simulink model "openMHA_test_ar_filter"  (R2020a)
settings: Solver=VariableStepAuto  StartTime=0.0  StopTime=stop_time  RelTol=1e-3
InitFcn:
  | test_ar_filter_init
StopFcn:
  | test_ar_filter_stop
values from neighbouring files (symbols this model uses):
  c1_a = exp( -1.0/(tau_a * fs) )    [test_FFT_to_gain_init.m]    (also in test_ar_filter_gaintable_init.m; test_ar_filter_init.m; test_db_ar_gaintable_init.m)
  c1_r = exp( -1.0/(tau_r * fs) )    [test_FFT_to_gain_init.m]    (also in test_ar_filter_gaintable_init.m; test_ar_filter_init.m; test_db_ar_gaintable_init.m)
  c2_a = 1.0 - c1_a    [test_FFT_to_gain_init.m]    (also in test_ar_filter_gaintable_init.m; test_ar_filter_init.m; test_db_ar_gaintable_init.m)
  c2_r = 1.0 - c1_r    [test_FFT_to_gain_init.m]    (also in test_ar_filter_gaintable_init.m; test_ar_filter_init.m; test_db_ar_gaintable_init.m)
libraries: simulink x1, dspsrcs4 x1
settings Model: PacingRate=112  Creator=t96f346  LastModifiedBy=t96f346

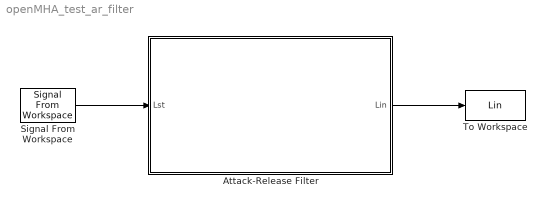
== system openMHA_test_ar_filter ==
  Attack-Release Filter : Subsystem
  Signal From Workspace : dspsrcs4/Signal From Workspace  X=Lst  Ts=1  nsamps=1  OutputAfterFinalValue=Setting to zero  ignoreOrWarnInputAndFrameLengths=off  OutputFrames=off
  To Workspace : ToWorkspace  VariableName=Lin  SampleTime=-1
      settings: Save2DSignal=2-D array (concatenate along first dimension)
  wires:
  Signal From Workspace/1 -> Attack-Release Filter/1(Lst)
  Attack-Release Filter/1(Lin) -> To Workspace/1

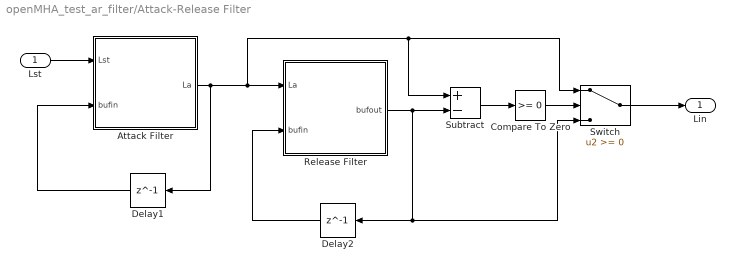
== system openMHA_test_ar_filter/Attack-Release Filter ==
  Lst : Inport
  Attack Filter : Subsystem  TreatAsAtomicUnit=on
  Compare To Zero : simulink/Logic and Bit Operations/Compare To Zero  relop=>=  OutDataTypeStr=boolean
  Delay1 : Delay  DelayLength=1  InitialCondition=65
  Delay2 : Delay  DelayLength=1  InitialCondition=65
  Release Filter : Subsystem  TreatAsAtomicUnit=on
  Subtract : Sum  Inputs=+-  OutDataTypeStr=Inherit: Same as accumulator
  Switch : Switch
  Lin : Outport  VectorParamsAs1DForOutWhenUnconnected=off
  wires:
  Lst/1 -> Attack Filter/1(Lst)
  Delay2/1 -> Release Filter/2(bufin)
  Delay1/1 -> Attack Filter/2(bufin)
  Subtract/1 -> Compare To Zero/1
  Switch/1 -> Lin/1
  Release Filter/1(bufout) -> Subtract/2, Delay2/1, Switch/3
  Compare To Zero/1 -> Switch/2
  Attack Filter/1(La) -> Delay1/1, Subtract/1, Switch/1, Release Filter/1(La)

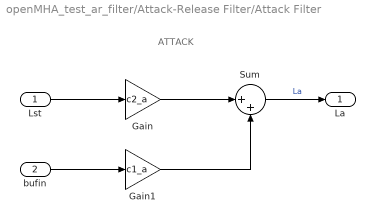
== system openMHA_test_ar_filter/Attack-Release Filter/Attack Filter ==
  note: ATTACK
  Lst : Inport
  bufin : Inport  Port=2
  Gain : Gain  Gain=c2_a
  Gain1 : Gain  Gain=c1_a
  Sum : Sum  Inputs=|++
  La : Outport  InitialOutput=0  VectorParamsAs1DForOutWhenUnconnected=off
  wires:
  Lst/1 -> Gain/1
  Gain/1 -> Sum/1
  Sum/1 -> La/1  "La"
  bufin/1 -> Gain1/1
  Gain1/1 -> Sum/2

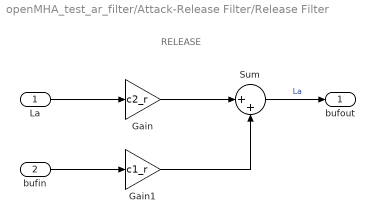
== system openMHA_test_ar_filter/Attack-Release Filter/Release Filter ==
  note: RELEASE
  La : Inport
  bufin : Inport  Port=2
  Gain : Gain  Gain=c2_r
  Gain1 : Gain  Gain=c1_r
  Sum : Sum  Inputs=|++
  bufout : Outport  InitialOutput=0  VectorParamsAs1DForOutWhenUnconnected=off
  wires:
  Sum/1 -> bufout/1  "La"
  Gain/1 -> Sum/1
  Gain1/1 -> Sum/2
  bufin/1 -> Gain1/1
  La/1 -> Gain/1
